simulink model "tfAfDamp"  (R2017b)
settings: Solver=VariableStepAuto  StartTime=0.0  StopTime=100.0  RelTol=1e-3
values from neighbouring files (symbols this model uses):
  Kp = 1/M    [Opgave33.m]    (also in tfAfDamp_konstanter.m)
  stepsize = 1    [tfAfDamp_konstanter.m]
  tau_i = Ni/omega_c    (= 0.46511627907)    [Opgave33.m]    (also in tfAfDamp_konstanter.m = 32.0512820513)
settings Model: Creator=asger  LastModifiedBy=tilfr

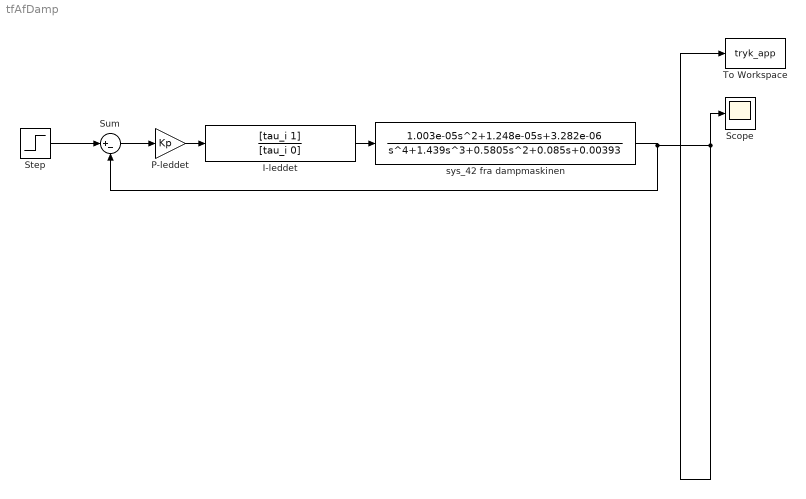
== system tfAfDamp ==
  I-leddet : TransferFcn  Numerator=[tau_i 1]  Denominator=[tau_i 0]
  P-leddet : Gain  Gain=Kp
  Scope : Scope
  Step : Step  Time=0  After=stepsize  SampleTime=0
  Sum : Sum  Inputs=|+-
  To Workspace : ToWorkspace  VariableName=tryk_app  SaveFormat=Timeseries  SampleTime=-1
  sys_42 fra dampmaskinen : TransferFcn  Numerator=[1.003e-05 1.248e-05 3.282e-06]  Denominator=[1 1.439 0.5805 0.085 0.00393]
  wires:
  sys_42 fra dampmaskinen/1 -> Sum/2, To Workspace/1, Scope/1
  Step/1 -> Sum/1
  Sum/1 -> P-leddet/1
  P-leddet/1 -> I-leddet/1
  I-leddet/1 -> sys_42 fra dampmaskinen/1
